simulink library "WECSim_Lib_Frames"  (R2020b)
settings: Solver=VariableStepAuto  StartTime=0.0  StopTime=10.0  RelTol=1e-3
undefined symbols (not defined in the file): simu, waves, X, Y, Z
libraries: sm_lib x8, nesl_utility x2
settings Model: Creator=kmruehl  LastModifiedBy=huangxuanrui
settings DebuggingCC: SFMachineParentedDataDiag=error

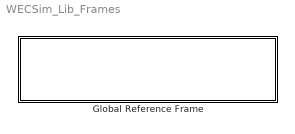
== system WECSim_Lib_Frames ==
  Global Reference Frame : Subsystem  mask(Frames){waves=waves, simu=simu, InputMethod=Input File, InputFile=wecSimInputFile.m, mode=normal, explorer=off, solver=ode4, startTime=0, rampTime=100, endTime=400, dt=0.1, cicEndTime=60, stateSpace=0, WaveClass=regular, height=2.5, period=8, elevationFile=NOT DEFINED, spectrumFile=NOT DEFINED, direction=0, spread=1, spectrumType=NOT DEFINED, phaseSeed=0, option=EqualEnergy}
      mask prompts: waves "Wave Class Name"; simu "Simulation Class Name"; InputMethod "Parameter Input Method"; mode "Simulation Mode:"; explorer "SimMechanics Explorer:"; solver "SimSolver:"; startTime "Start Time [s]:"; rampTime "Ramp Time [s]:"; endTime "End Time [s]:"; dt "Step Size [s]:"; cicEndTime "CI Time [s]:"; stateSpace "Turn on State Space"; WaveClass "Select Wave Class:"; height "Wave Height [m]:"; period "Wave Period [s]:"; direction "Wave Direction [deg]:"; spread "Wave Spread [0-1]:"; spectrumType "Wave Spectrum Type:"; phaseSeed "Phase Seed:"; option "Frequency Discretization:"
      mask help:
      | This block contains Global References, including solver configurations, free surface and seabed description, and simulation time.
      | It uses the following fields from the Simulation and Wave classes:
      |
      | Simulation Class:
      |     .endTime
      |     .dt
      |     .domainSize
      |
      | Wave Class:
      |     .waterDepth
      mask Help:
      | This block contains Global References, including solver configurations, free surface and seabed description, and simulation time.
      | It uses the following fields from the Simulation and Wave classes:
      | 
      | Simulation Class:
      |     .endTime
      |     .dt
      |     .domainSize
      | 
      | Wave Class:
      |     .waterDepth
      mask TypeOptions InputMethod: Input File | Custom Parameters
      mask Callback InputMethod: inputOrCustomCallback(gcbh)
      mask TypeOptions mode: normal | accelerator | rapid-accelerator
      mask TypeOptions explorer: on | off
      mask TypeOptions solver: ode4 | ode45
      mask TypeOptions stateSpace: 0 | 1
      mask TypeOptions WaveClass: noWaveCIC | regular | regularCIC | irregular | spectrumImport | etaImport
      mask Callback WaveClass: waveClassCallback(gcbh)
      mask TypeOptions spectrumType: PM | JS | NOT DEFINED
      mask TypeOptions option: EqualEnergy | Traditional
      mask DialogControl InputFileGroup Prompt: Input File
      mask DialogControl InFileButton Prompt: Select File
      mask DialogControl InFileButton Callback: inFileButtonCallback(gcbh)
      mask DialogControl CustomParameterGroup Prompt: Custom Parameters
      mask DialogControl LoadParam Prompt: Load parameters from Input File
      mask DialogControl LoadParam Callback: loadInputFileCallback(gcbh)
      mask DialogControl SimData Prompt: Simulation Data
      mask DialogControl WaveInfo Prompt: Wave Information
      mask DialogControl ETAbutton Prompt: Select etaData.mat file
      mask DialogControl ETAbutton Callback: etaButtonCallback(gcbh)
      mask DialogControl SpecButton Prompt: Select spectrumData.mat file
      mask DialogControl SpecButton Callback: spectrumButtonCallback(gcbh)
      mask Display: fprintf('Active Method: \n%s',get_param(gcbh,'InputMethod'))

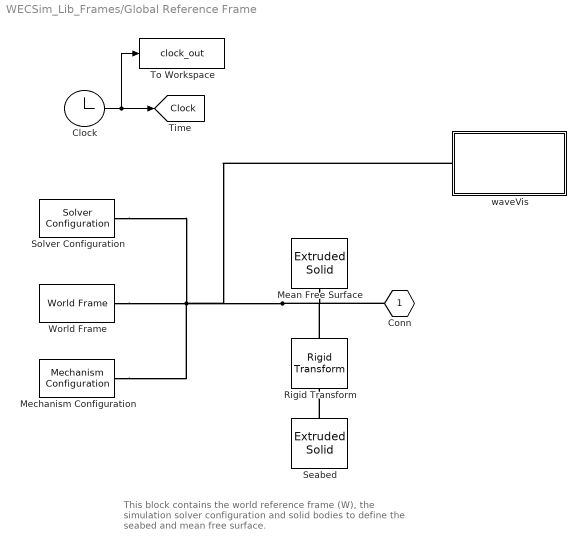
== system WECSim_Lib_Frames/Global Reference Frame ==
  note: This block contains the world reference frame (W), the simulation solver configuration and
      | solid bodies to define the seabed and mean free surface.
  Clock : Clock
  Mean Free Surface : sm_lib/Body Elements/Extruded Solid  GraphicAmbientColor=[0.15 0.15 0.15 1.0]  BasedOnType=Density  CenterOfMass=[0 0 0]  CenterOfMassUnits=m  GraphicDiffuseColor=[0.0 0.6 0.8]  ExportConvexHullGeometry=off  ExtrusionCrossSection=[simu.domainSize simu.domainSize; -simu.domainSize simu.domainSize; -simu.domainSize -simu.domainSize; simu.domainSize -simu.domainSize]  ExtrusionCrossSectionUnits=m  Density=1000  DensityUnits=kg/(m^3)  DoExposeReferenceFrame=on  GraphicEmissiveColor=[0.0 0.0 0.0 1.0]  ExportEntireGeometry=off  ExtrusionLength=simu.domainSize/200  ExtrusionLengthUnits=m  ExtrusionType=General  SerializedFrames=<Frames/>  MarkerShape=Sphere  MarkerSize=10  GraphicType=FromGeometry  InertiaType=Custom  Mass=10^20  MassUnits=kg  MomentsOfInertia=[10^20 10^20 10^20]  MomentsOfInertiaUnits=kg*m^2  PolygonNumSides=3  GraphicOpacity=0.3  PolygonOuterRadius=1  PolygonOuterRadiusUnits=m  ProductsOfInertia=[0 0 0]  ProductsOfInertiaUnits=kg*m^2  GraphicShininess=75  GraphicSpecularColor=[0.5 0.5 0.5 1.0]  GraphicVisPropType=SimpleVisualProperties
  Mechanism Configuration : sm_lib/Utilities/Mechanism Configuration  UniformGravity=Constant  GravityVector=[0 0 0]  GravityVectorUnits=m/s^2  GravityUnits=m/s^2  LinearizationDelta=0.001  JointModeTransitionNonlinearIterations=2
  Rigid Transform : sm_lib/Frames and Transforms/Rigid Transform  TranslationMethod=Cartesian  TranslationStandardOffset=0  TranslationLengthUnit=m  TranslationStandardAxis=+Z  TranslationCartesianOffset=[0 0 -waves.waterDepth]  TranslationROffset=0  TranslationROffsetUnits=m  TranslationZOffset=0  TranslationZOffsetUnits=m  TranslationThetaOffset=0  TranslationThetaOffsetUnits=deg  RotationMethod=None  RotationAngleUnits=deg  RotationStandardAxis=+Z  RotationAngle=0  RotationArbitraryAxis=[0 0 1]  FollAlignAxisA=+X  BaseAlignAxisA=+Y  FollAlignAxisB=+Y  BaseAlignAxisB=+Z  RotationSequenceAxes=FollowerAxes  RotationSequence=XYX  RotationSequenceAngles=[0 0 0]  RotationSequenceAnglesUnits=deg  RotationMatrix=[1 0 0; 0 1 0; 0 0 1]
  Seabed : sm_lib/Body Elements/Extruded Solid  GraphicAmbientColor=[0.15 0.15 0.15 1.0]  BasedOnType=Density  CenterOfMass=[0 0 0]  CenterOfMassUnits=m  GraphicDiffuseColor=[0.4 0.4 0.0]  ExportConvexHullGeometry=off  ExtrusionCrossSection=[simu.domainSize simu.domainSize; -simu.domainSize simu.domainSize; -simu.domainSize -simu.domainSize; simu.domainSize -simu.domainSize]  ExtrusionCrossSectionUnits=m  Density=1000  DensityUnits=kg/(m^3)  DoExposeReferenceFrame=on  GraphicEmissiveColor=[0.0 0.0 0.0 1.0]  ExportEntireGeometry=off  ExtrusionLength=simu.domainSize/100  ExtrusionLengthUnits=m  ExtrusionType=General  SerializedFrames=<Frames/>  MarkerShape=Sphere  MarkerSize=10  GraphicType=FromGeometry  InertiaType=Custom  Mass=10^20  MassUnits=kg  MomentsOfInertia=[10^20 10^20 10^20]  MomentsOfInertiaUnits=kg*m^2  PolygonNumSides=3  GraphicOpacity=1  PolygonOuterRadius=1  PolygonOuterRadiusUnits=m  ProductsOfInertia=[0 0 0]  ProductsOfInertiaUnits=kg*m^2  GraphicShininess=75  GraphicSpecularColor=[0.5 0.5 0.5 1.0]  GraphicVisPropType=SimpleVisualProperties
  Solver Configuration : nesl_utility/Solver Configuration  PhysicalDomain=network_engine_domain  SubClassName=solver  LeftPortType=input  RightPortType=generic  Tones=[]  Harmonics=[]  SimulateNoise=off  Profile=off  UseLocalSampling=off  EnableSwitchedLinearOptims=on  FrequencyDomain=off  UseCCode=off  RelTol=0.001  AbsTol=1e-06  MinStep=1e-09  ToWorkspace=off  RevertToSquareIcSolve=off  NumHomotopyIterations=100  PhasorMode=off  PhasorModeNumHarmonics=1  DoDC=on  ResidualTolerance=1e-9  UseLocalSolver=off  LocalSolverChoice=NE_BACKWARD_EULER_ADVANCER  LocalSolverSampleTime=.001  DoFixedCost=off  MaxNonlinIter=3  MaxModeIter=2  ComputeImpulses=off  ImpulseIterations=2  LinearAlgebra=Sparse  EquationFormulation=NE_TIME_EF  DelaysMemoryBudget=1024  AutomaticFiltering=on  FilteringTimeConstant=0.001  PartitionStorageMethod=AS_NEEDED  PartitionMemoryBudget=1024  PartitionMethod=FAST
      settings: SourceProductBaseCode=PW,SS
  To Workspace : ToWorkspace  VariableName=clock_out  SaveFormat=Structure With Time  SampleTime=-1
  World Frame : sm_lib/Frames and Transforms/World Frame
  waveVis : Subsystem  Variant=on  VariantControl=Choice  AllowZeroVariantControls=on  PropagateVariantConditions=on  mask{visualizationON=0}
      mask prompts: visualizationON "Visualization Option"
      mask init:
      | % sv_visulizationON  =Simulink.Variant('visualizationON');
      | % sv_visulizationOFF =Simulink.Variant('visualizationOFF');
      | 
      |     h = [gcb '/waveVisOff'];
      |     visualizationON = 'sv_visualizationOFF';
      |     set_param(h,'VariantControl',visualizationON);
      |     
      |     h = [gcb '/waveVisOn'];
      |     visualizationON = 'sv_visualizationON';
      |     set_param(h,'VariantControl',visualizationON);
      mask TypeOptions visualizationON: 0  | 1
  Conn : PMIOPort  Side=Right
  tag scope: Clock=global
  wires:
  Clock/1 -> To Workspace/1, [Clock]
  connections:
  World Frame/RConn1 -- Mechanism Configuration/RConn1 -- waveVis/LConn1 -- Conn/RConn1 -- Mean Free Surface/RConn1 -- Rigid Transform/LConn1 -- Solver Configuration/RConn1
  Seabed/RConn1 -- Rigid Transform/RConn1

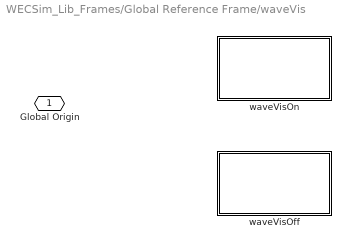
== system WECSim_Lib_Frames/Global Reference Frame/waveVis ==
  waveVisOff : Subsystem  VariantControl=sv_visualizationOFF
  waveVisOn : Subsystem  VariantControl=sv_visualizationON
  Global Origin : PMIOPort  Side=Left

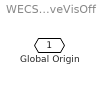
== system WECSim_Lib_Frames/Global Reference Frame/waveVis/waveVisOff ==
  Global Origin : PMIOPort  Side=Left

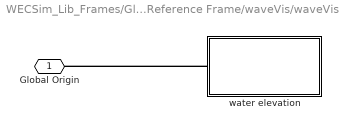
== system WECSim_Lib_Frames/Global Reference Frame/waveVis/waveVisOn ==
  water elevation : Subsystem  mask{waves=waves, wgloc=0, wgT=0}
      mask prompts: waves "Waves Object"; wgloc "Waves Gauge Location [X,Y]"; wgT "Waves Gauge Time History"
      mask init:
      | cb = gcb;
      | 
      | set_param([cb '/marker1'],...
      |            'position',[0,100,180,140]);
      | set_param([cb '/marker1'],...
      |            'wgloc',[sprintf('waves.marker.location(%d,:)',1)]); 
      | set_param([cb '/marker1'],...
      |            'wgT',[sprintf('[waves.waveAmpTimeViz(:,1), waves.waveAmpTimeViz(:,%d)]',2)]);
      | 
      | nGauges = size(waves.marker.location,1);
      | for iWG = 2:nGauges
      |     try 
      |         find_system([cb,'/marker',num2str(iWG)],'Type','Block');
      |     catch
      |         add_block([cb,'/marker1'],[cb,'/marker',num2str(iWG)],'MakeNameUnique','off',...
      |                    'Position',[0,100*iWG,180,40+100*iWG],'BackgroundColor','white');
      |         set_param([cb,'/marker',num2str(iWG)],'wgT',[sprintf('[waves.waveAmpTimeViz(:,1),waves.waveAmpTimeViz(:,%d)]',iWG+1)]);
      |         set_param([cb,'/marker',num2str(iWG)],'wgloc',[sprintf('waves.marker.location(%d,:)',iWG)]);
      |         add_line(cb,...
      |             ['marker',num2str(iWG),'/LConn1'],...
      |             ['Global Origin/RConn1'],...
      |             'autorouting','on');
      |     end
      | end
  Global Origin : PMIOPort  Side=Left
  connections:
  water elevation/LConn1 -- Global Origin/RConn1

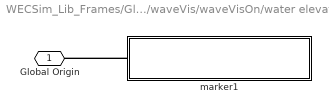
== system WECSim_Lib_Frames/Global Reference Frame/waveVis/waveVisOn/water elevation ==
  marker1 : Subsystem  mask{wgloc=waves.marker.location(1,:), wgT=[waves.waveAmpTimeViz(:,1), waves.waveAmpTimeViz(:,2)]}
      mask prompts: wgloc "Wave Gauge Location [X,Y]"; wgT "Wave Gauge Time History"
  Global Origin : PMIOPort  Side=Left
  connections:
  marker1/LConn1 -- Global Origin/RConn1

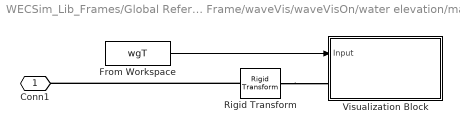
== system WECSim_Lib_Frames/Global Reference Frame/waveVis/waveVisOn/water elevation/marker1 ==
  From Workspace : FromWorkspace  VariableName=wgT
  Rigid Transform : sm_lib/Frames and Transforms/Rigid Transform  TranslationMethod=Cartesian  TranslationStandardOffset=0  TranslationLengthUnit=m  TranslationStandardAxis=+Z  TranslationCartesianOffset=[wgloc 0]  TranslationROffset=0  TranslationROffsetUnits=m  TranslationZOffset=0  TranslationZOffsetUnits=m  TranslationThetaOffset=0  TranslationThetaOffsetUnits=deg  RotationMethod=None  RotationAngleUnits=deg  RotationStandardAxis=+Z  RotationAngle=0.0  RotationArbitraryAxis=[0 0 1]  FollAlignAxisA=+X  BaseAlignAxisA=+Y  FollAlignAxisB=+Y  BaseAlignAxisB=+Z  RotationSequenceAxes=FollowerAxes  RotationSequence=XYX  RotationSequenceAngles=[0 0 0]  RotationSequenceAnglesUnits=deg  RotationMatrix=[1 0 0; 0 1 0; 0 0 1]
  Visualization Block : Subsystem  mask{markStyle=waves.marker.style, markSize=waves.marker.size}
      mask prompts: markStyle "Waves Marker Style"; markSize "Waves Marker Size"
      mask init:
      | % Marker Shape %<MarkerShape>
      | % Marker Size %<MarkerSize>%<MarkerSizeUnits>
      | cb = gcb;
      | 
      | set_param([cb '/WaveElevation'],'MarkerSize','markSize')
      | 
      | if markStyle == 1
      |     set_param([cb '/WaveElevation'],'MarkerShape','Sphere')
      | elseif markStyle == 2
      |     set_param([cb '/WaveElevation'],'MarkerShape','Cube')
      | elseif markStyle == 3
      |     set_param([cb '/WaveElevation'],'MarkerShape','Frame')
      | end
  Conn1 : PMIOPort  Side=Left
  wires:
  From Workspace/1 -> Visualization Block/1(Input)
  connections:
  Rigid Transform/RConn1 -- Visualization Block/LConn1
  Rigid Transform/LConn1 -- Conn1/RConn1

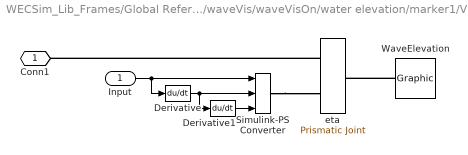
== system WECSim_Lib_Frames/Global Reference Frame/waveVis/waveVisOn/water elevation/marker1/Visualization Block ==
  Input : Inport
  Derivative : Derivative
  Derivative1 : Derivative
  Simulink-PS Converter : nesl_utility/Simulink-PS Converter  PhysicalDomain=network_engine_domain  SubClassName=ps_input  LeftPortType=input  RightPortType=output  PseudoPeriodic=off  Frequencies=[]  NoiseDistribution=none  NoiseParameters=[]  Unit=1  AffineConversion=off  FilteringAndDerivatives=provide  SimscapeFilterOrder=1  InputFilterTimeConstant=0.001  UdotUserProvided=2
      settings: SourceProductBaseCode=PW,SS
  WaveElevation : sm_lib/Body Elements/Graphic  GraphicType=Marker  MarkerShape=Sphere  MarkerSize=markSize  GraphicVisPropType=SimpleVisualProperties  GraphicDiffuseColor=[0.2 1.0 0.6]  GraphicSpecularColor=[0.5 0.5 0.5 1.0]  GraphicAmbientColor=[0.15 0.15 0.15 1.0]  GraphicEmissiveColor=[0.0 0.0 0.0 1.0]  GraphicShininess=75  GraphicOpacity=1.0
      settings: AttributesFormatString=|
      | Marker Shape: %<MarkerShape>
      | Marker Size:    %<MarkerSize>%<MarkerSizeUnits>
  eta : sm_lib/Joints/Prismatic Joint  JointMode=Normal  SenseConstraintForce=off  SenseConstraintForceX=off  SenseConstraintForceY=off  SenseConstraintForceZ=off  SenseConstraintTorque=off  SenseConstraintTorqueX=off  SenseConstraintTorqueY=off  SenseConstraintTorqueZ=off  SenseTotalForce=off  SenseTotalForceX=off  SenseTotalForceY=off  SenseTotalForceZ=off  SenseTotalTorque=off  SenseTotalTorqueX=off  SenseTotalTorqueY=off  SenseTotalTorqueZ=off  CompositeWrenchDir=FollowerOnBase  CompositeWrenchFrame=BaseFrame  EquilibriumPosition=0  EquilibriumPositionUnits=m  SpringStiffness=0  SpringStiffnessUnits=N/m  DampingCoefficient=0  DampingCoefficientUnits=N/(m/s)  TorqueActuationMode=ComputedTorque  MotionActuationMode=InputMotion  SensePosition=off  SenseVelocity=off  SenseAcceleration=off  SenseTorqueForce=off  SenseLowerLimitTorqueForce=off  SenseUpperLimitTorqueForce=off  LowerLimitSpecify=off  LowerLimitBound=-1  LowerLimitBoundUnits=m  LowerLimitStiffness=1e6  LowerLimitStiffnessUnits=N/m  LowerLimitDamping=1e3  LowerLimitDampingUnits=N/(m/s)  LowerLimitTransitionRegionWidth=1e-4  LowerLimitTransitionRegionWidthUnits=m  UpperLimitSpecify=off  UpperLimitBound=1  UpperLimitBoundUnits=m  UpperLimitStiffness=1e6  UpperLimitStiffnessUnits=N/m  UpperLimitDamping=1e3  UpperLimitDampingUnits=N/(m/s)  UpperLimitTransitionRegionWidth=1e-4  UpperLimitTransitionRegionWidthUnits=m  PositionTargetSpecify=off  PositionTargetPriority=High  PositionTargetValue=0  PositionTargetValueUnits=m  VelocityTargetSpecify=off  VelocityTargetPriority=High  VelocityTargetValue=0  VelocityTargetValueUnits=m/s
  Conn1 : PMIOPort  Side=Left
  wires:
  Input/1 -> Derivative/1, Simulink-PS Converter/1
  Derivative/1 -> Derivative1/1, Simulink-PS Converter/2
  Derivative1/1 -> Simulink-PS Converter/3
  connections:
  Simulink-PS Converter/RConn1 -- eta/LConn2
  WaveElevation/RConn1 -- eta/RConn1
  eta/LConn1 -- Conn1/RConn1
